simulink model "EventDrivenSimulationModel"  (R2023b)
settings: Solver=VariableStepAuto  StartTime=0.0  StopTime=ModelingDur  RelTol=1e-3  EnableMultiTasking=on
undefined symbols (not defined in the file): m, n
settings Model: Creator=The MathWorks, Inc.  LastModifiedBy=paulius
settings SolverCC: AlgebraicLoopSolver=TrustRegion
settings DataIOCC: LimitDataPoints=on  SaveFormat=Array  ReturnWorkspaceOutputs=off
settings OptimizationCC: LifeSpan=inf
settings DebuggingCC: UnconnectedInputMsg=warning  UnconnectedOutputMsg=warning  UnconnectedLineMsg=warning  AllowSymbolicDim=off  SFUnexpectedBacktrackingDiag=warning  SFNoUnconditionalDefaultTransitionDiag=warning  SFExecutionAtInitializationDiag=none  ArithmeticOperatorsInVariantConditions=warning
settings ModelReferenceCC: EnableRefExpFcnMdlSchedulingChecks=on  PropagateSignalLabelsOutOfModel=off
settings SFSimCC: SimUseLocalCustomCode=off  CustomCodeUndefinedFunction=UseInterfaceOnly
settings RTWCC: RTWUseLocalCustomCode=off  DLArmComputeVersion=19.05
settings CodeAppCC: StateflowObjectComments=on
settings GRTTargetCC: TargetLangStandard=C89/C90 (ANSI)
settings ConfigComp: CovMetricSettings=dw  CovSaveCumulativeToWorkspaceVar=on  CovSaveSingleToWorkspaceVar=on  CovExternalEMLEnable=off  CovSFcnEnable=off

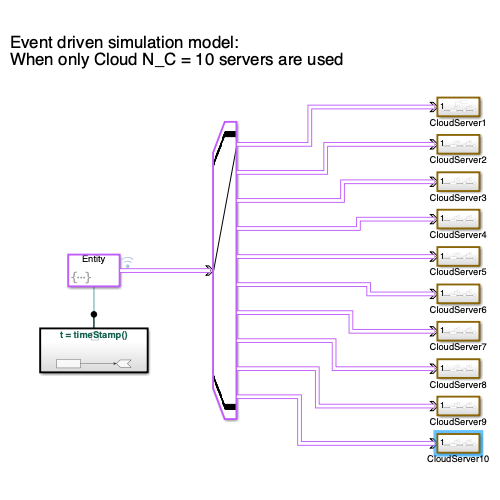
[thumbnail: Simulink's stored preview of the top-level diagram]
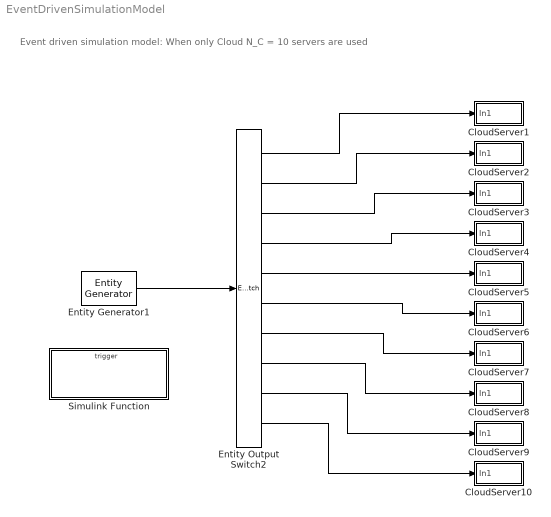
== system EventDrivenSimulationModel ==
  note: Event driven simulation model:
      | When only Cloud N_C = 10 servers are used
  CloudServer1 : Subsystem
  CloudServer10 : Subsystem
  CloudServer2 : Subsystem
  CloudServer3 : Subsystem
  CloudServer4 : Subsystem
  CloudServer5 : Subsystem
  CloudServer6 : Subsystem
  CloudServer7 : Subsystem
  CloudServer8 : Subsystem
  CloudServer9 : Subsystem
  Entity Output Switch2 : EntityOutputSwitch  InputPortMessageModes=m  OutputPortMessageModes=m,m,m,m,m,m,m,m,m,m  NumberOutputPorts=10  SwitchingCriterion=From attribute  SwitchAttributeName=cloud_server_no
      settings: OutputPortMap=o0,o1,o2,o3,o4,o5,o6,o7,o8,o9
  Entity Generator1 : EntityGenerator  OutputPortMessageModes=m  TimeSource=MATLAB action  IntergenerationTimeAction=|  GenerateAction=entity.cloud_server_no = randi(10);  AttributeName=Attribute1|proc_dest|edge_no|cloud_server_no|qsys  AttributeInitialValue=1|1|1|1|1  EntityType=Structured  EntityTypeName=Entity
      | t = timeStamp();
      | 
      | dtvid = 1/lambda; % vid laikotarpis tarp matavimu [h]
      | % kai Puasono (paprastasis) srautas - dt pagael exp skirstini
      | dt = -dtvid * log(1 - rand());
  Simulink Function : Subsystem  TreatAsAtomicUnit=on
  wires:
  Entity Generator1/1 -> Entity Output Switch2/1
  Entity Output Switch2/1 -> CloudServer1/1(In1)
  Entity Output Switch2/2 -> CloudServer2/1(In1)
  Entity Output Switch2/3 -> CloudServer3/1(In1)
  Entity Output Switch2/4 -> CloudServer4/1(In1)
  Entity Output Switch2/5 -> CloudServer5/1(In1)
  Entity Output Switch2/6 -> CloudServer6/1(In1)
  Entity Output Switch2/7 -> CloudServer7/1(In1)
  Entity Output Switch2/8 -> CloudServer8/1(In1)
  Entity Output Switch2/9 -> CloudServer9/1(In1)
  Entity Output Switch2/10 -> CloudServer10/1(In1)

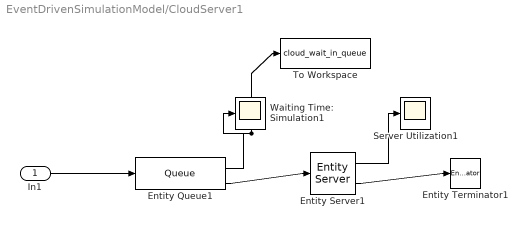
== system EventDrivenSimulationModel/CloudServer1 ==
  In1 : Inport
  Entity Queue1 : Queue  InputPortMessageModes=m  OutputPortMessageModes=n,m  Capacity=Inf  AverageWait=on
      settings: OutputPortMap=o2,o5
  Entity Server1 : EntityServer  InputPortMessageModes=m  OutputPortMessageModes=n,m  Capacity=1  ServiceTimeSource=MATLAB action  ServiceTimeAction=|  Utilization=on
      | if qsys == 1 % 'mm1' exponential T_C distribution
      |     dt = -mean_T_C * log(1 - rand()); 
      | elseif qsys == 2 % 'mg1' - general (normal) T_C distribution
      |     dt = mean_T_C+std_T_C*randn();
      |     if dt < 0
      |         dt = 0;
      |     end
      | else % 'md1' - deterministic (const.) T_C distribution
      |     dt = mean_T_C; 
      | end
      settings: OutputPortMap=o5,o9
  Entity Terminator1 : EntityTerminator  InputPortMessageModes=m
  Server Utilization1 : Scope
  To Workspace : ToWorkspace  VariableName=cloud_wait_in_queue  SaveFormat=Timeseries  SampleTime=-1
  Waiting Time: Simulation1 : Scope
  wires:
  Entity Server1/2 -> Entity Terminator1/1
  Entity Queue1/2 -> Entity Server1/1
  In1/1 -> Entity Queue1/1
  Entity Queue1/1 -> To Workspace/1, Waiting Time: Simulation1/1
  Entity Server1/1 -> Server Utilization1/1

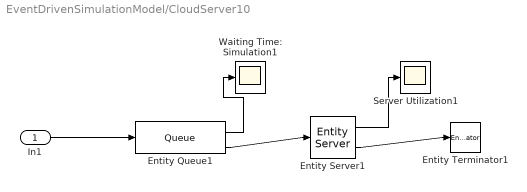
== system EventDrivenSimulationModel/CloudServer10 ==
  In1 : Inport
  Entity Queue1 : Queue  InputPortMessageModes=m  OutputPortMessageModes=n,m  Capacity=Inf  AverageWait=on
      settings: OutputPortMap=o2,o5
  Entity Server1 : EntityServer  InputPortMessageModes=m  OutputPortMessageModes=n,m  Capacity=1  ServiceTimeSource=MATLAB action  ServiceTimeAction=|  Utilization=on
      | if qsys == 1 % 'mm1' exponential T_C distribution
      |     dt = -mean_T_C * log(1 - rand()); 
      | elseif qsys == 2 % 'mg1' - general (normal) T_C distribution
      |     dt = mean_T_C+std_T_C*randn();
      |     if dt < 0
      |         dt = 0;
      |     end
      | else % 'md1' - deterministic (const.) T_C distribution
      |     dt = mean_T_C; 
      | end
      settings: OutputPortMap=o5,o9
  Entity Terminator1 : EntityTerminator  InputPortMessageModes=m
  Server Utilization1 : Scope
  Waiting Time: Simulation1 : Scope
  wires:
  Entity Server1/2 -> Entity Terminator1/1
  Entity Queue1/2 -> Entity Server1/1
  In1/1 -> Entity Queue1/1
  Entity Queue1/1 -> Waiting Time: Simulation1/1
  Entity Server1/1 -> Server Utilization1/1

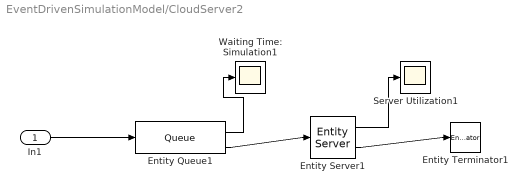
== system EventDrivenSimulationModel/CloudServer2 ==
  In1 : Inport
  Entity Queue1 : Queue  InputPortMessageModes=m  OutputPortMessageModes=n,m  Capacity=Inf  AverageWait=on
      settings: OutputPortMap=o2,o5
  Entity Server1 : EntityServer  InputPortMessageModes=m  OutputPortMessageModes=n,m  Capacity=1  ServiceTimeSource=MATLAB action  ServiceTimeAction=|  Utilization=on
      | if qsys == 1 % 'mm1' exponential T_C distribution
      |     dt = -mean_T_C * log(1 - rand()); 
      | elseif qsys == 2 % 'mg1' - general (normal) T_C distribution
      |     dt = mean_T_C+std_T_C*randn();
      |     if dt < 0
      |         dt = 0;
      |     end
      | else % 'md1' - deterministic (const.) T_C distribution
      |     dt = mean_T_C; 
      | end
      settings: OutputPortMap=o5,o9
  Entity Terminator1 : EntityTerminator  InputPortMessageModes=m
  Server Utilization1 : Scope
  Waiting Time: Simulation1 : Scope
  wires:
  Entity Server1/2 -> Entity Terminator1/1
  Entity Queue1/2 -> Entity Server1/1
  In1/1 -> Entity Queue1/1
  Entity Queue1/1 -> Waiting Time: Simulation1/1
  Entity Server1/1 -> Server Utilization1/1

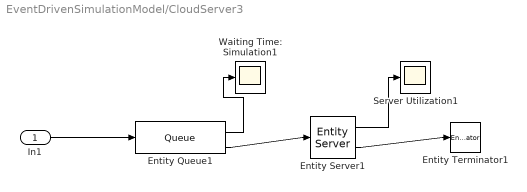
== system EventDrivenSimulationModel/CloudServer3 ==
  In1 : Inport
  Entity Queue1 : Queue  InputPortMessageModes=m  OutputPortMessageModes=n,m  Capacity=Inf  AverageWait=on
      settings: OutputPortMap=o2,o5
  Entity Server1 : EntityServer  InputPortMessageModes=m  OutputPortMessageModes=n,m  Capacity=1  ServiceTimeSource=MATLAB action  ServiceTimeAction=|  Utilization=on
      | if qsys == 1 % 'mm1' exponential T_C distribution
      |     dt = -mean_T_C * log(1 - rand()); 
      | elseif qsys == 2 % 'mg1' - general (normal) T_C distribution
      |     dt = mean_T_C+std_T_C*randn();
      |     if dt < 0
      |         dt = 0;
      |     end
      | else % 'md1' - deterministic (const.) T_C distribution
      |     dt = mean_T_C; 
      | end
      settings: OutputPortMap=o5,o9
  Entity Terminator1 : EntityTerminator  InputPortMessageModes=m
  Server Utilization1 : Scope
  Waiting Time: Simulation1 : Scope
  wires:
  Entity Server1/2 -> Entity Terminator1/1
  Entity Queue1/2 -> Entity Server1/1
  In1/1 -> Entity Queue1/1
  Entity Queue1/1 -> Waiting Time: Simulation1/1
  Entity Server1/1 -> Server Utilization1/1

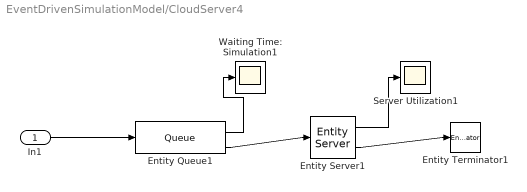
== system EventDrivenSimulationModel/CloudServer4 ==
  In1 : Inport
  Entity Queue1 : Queue  InputPortMessageModes=m  OutputPortMessageModes=n,m  Capacity=Inf  AverageWait=on
      settings: OutputPortMap=o2,o5
  Entity Server1 : EntityServer  InputPortMessageModes=m  OutputPortMessageModes=n,m  Capacity=1  ServiceTimeSource=MATLAB action  ServiceTimeAction=|  Utilization=on
      | if qsys == 1 % 'mm1' exponential T_C distribution
      |     dt = -mean_T_C * log(1 - rand()); 
      | elseif qsys == 2 % 'mg1' - general (normal) T_C distribution
      |     dt = mean_T_C+std_T_C*randn();
      |     if dt < 0
      |         dt = 0;
      |     end
      | else % 'md1' - deterministic (const.) T_C distribution
      |     dt = mean_T_C; 
      | end
      settings: OutputPortMap=o5,o9
  Entity Terminator1 : EntityTerminator  InputPortMessageModes=m
  Server Utilization1 : Scope
  Waiting Time: Simulation1 : Scope
  wires:
  Entity Server1/2 -> Entity Terminator1/1
  Entity Queue1/2 -> Entity Server1/1
  In1/1 -> Entity Queue1/1
  Entity Queue1/1 -> Waiting Time: Simulation1/1
  Entity Server1/1 -> Server Utilization1/1

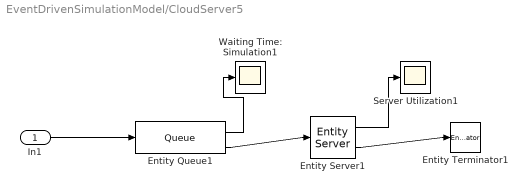
== system EventDrivenSimulationModel/CloudServer5 ==
  In1 : Inport
  Entity Queue1 : Queue  InputPortMessageModes=m  OutputPortMessageModes=n,m  Capacity=Inf  AverageWait=on
      settings: OutputPortMap=o2,o5
  Entity Server1 : EntityServer  InputPortMessageModes=m  OutputPortMessageModes=n,m  Capacity=1  ServiceTimeSource=MATLAB action  ServiceTimeAction=|  Utilization=on
      | if qsys == 1 % 'mm1' exponential T_C distribution
      |     dt = -mean_T_C * log(1 - rand()); 
      | elseif qsys == 2 % 'mg1' - general (normal) T_C distribution
      |     dt = mean_T_C+std_T_C*randn();
      |     if dt < 0
      |         dt = 0;
      |     end
      | else % 'md1' - deterministic (const.) T_C distribution
      |     dt = mean_T_C; 
      | end
      settings: OutputPortMap=o5,o9
  Entity Terminator1 : EntityTerminator  InputPortMessageModes=m
  Server Utilization1 : Scope
  Waiting Time: Simulation1 : Scope
  wires:
  Entity Server1/2 -> Entity Terminator1/1
  Entity Queue1/2 -> Entity Server1/1
  In1/1 -> Entity Queue1/1
  Entity Queue1/1 -> Waiting Time: Simulation1/1
  Entity Server1/1 -> Server Utilization1/1

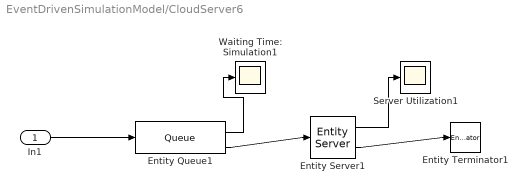
== system EventDrivenSimulationModel/CloudServer6 ==
  In1 : Inport
  Entity Queue1 : Queue  InputPortMessageModes=m  OutputPortMessageModes=n,m  Capacity=Inf  AverageWait=on
      settings: OutputPortMap=o2,o5
  Entity Server1 : EntityServer  InputPortMessageModes=m  OutputPortMessageModes=n,m  Capacity=1  ServiceTimeSource=MATLAB action  ServiceTimeAction=|  Utilization=on
      | if qsys == 1 % 'mm1' exponential T_C distribution
      |     dt = -mean_T_C * log(1 - rand()); 
      | elseif qsys == 2 % 'mg1' - general (normal) T_C distribution
      |     dt = mean_T_C+std_T_C*randn();
      |     if dt < 0
      |         dt = 0;
      |     end
      | else % 'md1' - deterministic (const.) T_C distribution
      |     dt = mean_T_C; 
      | end
      settings: OutputPortMap=o5,o9
  Entity Terminator1 : EntityTerminator  InputPortMessageModes=m
  Server Utilization1 : Scope
  Waiting Time: Simulation1 : Scope
  wires:
  Entity Server1/2 -> Entity Terminator1/1
  Entity Queue1/2 -> Entity Server1/1
  In1/1 -> Entity Queue1/1
  Entity Queue1/1 -> Waiting Time: Simulation1/1
  Entity Server1/1 -> Server Utilization1/1

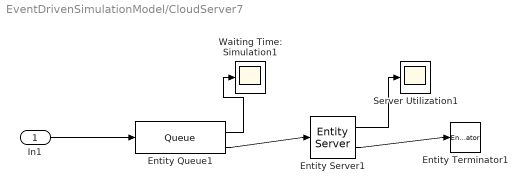
== system EventDrivenSimulationModel/CloudServer7 ==
  In1 : Inport
  Entity Queue1 : Queue  InputPortMessageModes=m  OutputPortMessageModes=n,m  Capacity=Inf  AverageWait=on
      settings: OutputPortMap=o2,o5
  Entity Server1 : EntityServer  InputPortMessageModes=m  OutputPortMessageModes=n,m  Capacity=1  ServiceTimeSource=MATLAB action  ServiceTimeAction=|  Utilization=on
      | if qsys == 1 % 'mm1' exponential T_C distribution
      |     dt = -mean_T_C * log(1 - rand()); 
      | elseif qsys == 2 % 'mg1' - general (normal) T_C distribution
      |     dt = mean_T_C+std_T_C*randn();
      |     if dt < 0
      |         dt = 0;
      |     end
      | else % 'md1' - deterministic (const.) T_C distribution
      |     dt = mean_T_C; 
      | end
      settings: OutputPortMap=o5,o9
  Entity Terminator1 : EntityTerminator  InputPortMessageModes=m
  Server Utilization1 : Scope
  Waiting Time: Simulation1 : Scope
  wires:
  Entity Server1/2 -> Entity Terminator1/1
  Entity Queue1/2 -> Entity Server1/1
  In1/1 -> Entity Queue1/1
  Entity Queue1/1 -> Waiting Time: Simulation1/1
  Entity Server1/1 -> Server Utilization1/1

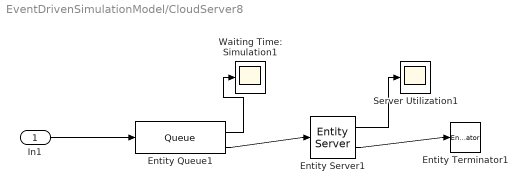
== system EventDrivenSimulationModel/CloudServer8 ==
  In1 : Inport
  Entity Queue1 : Queue  InputPortMessageModes=m  OutputPortMessageModes=n,m  Capacity=Inf  AverageWait=on
      settings: OutputPortMap=o2,o5
  Entity Server1 : EntityServer  InputPortMessageModes=m  OutputPortMessageModes=n,m  Capacity=1  ServiceTimeSource=MATLAB action  ServiceTimeAction=|  Utilization=on
      | if qsys == 1 % 'mm1' exponential T_C distribution
      |     dt = -mean_T_C * log(1 - rand()); 
      | elseif qsys == 2 % 'mg1' - general (normal) T_C distribution
      |     dt = mean_T_C+std_T_C*randn();
      |     if dt < 0
      |         dt = 0;
      |     end
      | else % 'md1' - deterministic (const.) T_C distribution
      |     dt = mean_T_C; 
      | end
      settings: OutputPortMap=o5,o9
  Entity Terminator1 : EntityTerminator  InputPortMessageModes=m
  Server Utilization1 : Scope
  Waiting Time: Simulation1 : Scope
  wires:
  Entity Server1/2 -> Entity Terminator1/1
  Entity Queue1/2 -> Entity Server1/1
  In1/1 -> Entity Queue1/1
  Entity Queue1/1 -> Waiting Time: Simulation1/1
  Entity Server1/1 -> Server Utilization1/1

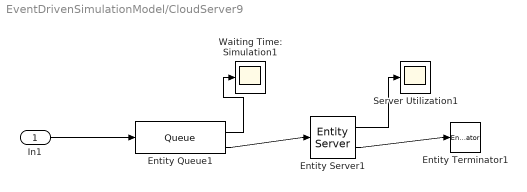
== system EventDrivenSimulationModel/CloudServer9 ==
  In1 : Inport
  Entity Queue1 : Queue  InputPortMessageModes=m  OutputPortMessageModes=n,m  Capacity=Inf  AverageWait=on
      settings: OutputPortMap=o2,o5
  Entity Server1 : EntityServer  InputPortMessageModes=m  OutputPortMessageModes=n,m  Capacity=1  ServiceTimeSource=MATLAB action  ServiceTimeAction=|  Utilization=on
      | if qsys == 1 % 'mm1' exponential T_C distribution
      |     dt = -mean_T_C * log(1 - rand()); 
      | elseif qsys == 2 % 'mg1' - general (normal) T_C distribution
      |     dt = mean_T_C+std_T_C*randn();
      |     if dt < 0
      |         dt = 0;
      |     end
      | else % 'md1' - deterministic (const.) T_C distribution
      |     dt = mean_T_C; 
      | end
      settings: OutputPortMap=o5,o9
  Entity Terminator1 : EntityTerminator  InputPortMessageModes=m
  Server Utilization1 : Scope
  Waiting Time: Simulation1 : Scope
  wires:
  Entity Server1/2 -> Entity Terminator1/1
  Entity Queue1/2 -> Entity Server1/1
  In1/1 -> Entity Queue1/1
  Entity Queue1/1 -> Waiting Time: Simulation1/1
  Entity Server1/1 -> Server Utilization1/1

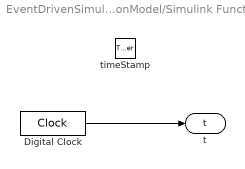
== system EventDrivenSimulationModel/Simulink Function ==
  timeStamp : TriggerPort  TriggerType=function-call  IsSimulinkFunction=on  FunctionName=timeStamp  FunctionVisibility=scoped  VariantControl=(inherit)
  Digital Clock : DigitalClock  SampleTime=-1
  t : ArgOut  DisableCoverage=on  ArgumentName=t
  wires:
  Digital Clock/1 -> t/1
